simulink model "enabledSin"  (R2017a)
settings: Solver=VariableStepAuto  StartTime=0.0  StopTime=10.0  RelTol=1e-3
libraries: simulink x2
settings Model: Creator=eruffaldi  LastModifiedBy=eruffaldi

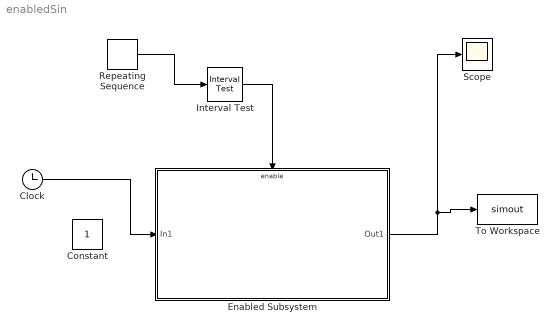
== system enabledSin ==
  Clock : Clock
  Constant : Constant
  Enabled Subsystem : Subsystem  TreatAsAtomicUnit=on
  Interval Test : simulink/Logic and Bit Operations/Interval Test  IntervalClosedRight=on  uplimit=3  IntervalClosedLeft=on  lowlimit=1  OutDataTypeStr=boolean
  Repeating Sequence : simulink/Sources/Repeating Sequence  rep_seq_t=[0 2 3]  rep_seq_y=[0 2 5]
  Scope : Scope
  To Workspace : ToWorkspace  VariableName=simout  SaveFormat=Timeseries  SampleTime=-1
  wires:
  Interval Test/1 -> Enabled Subsystem/Enable
  Repeating Sequence/1 -> Interval Test/1
  Enabled Subsystem/1(Out1) -> To Workspace/1, Scope/1
  Clock/1 -> Enabled Subsystem/1(In1)

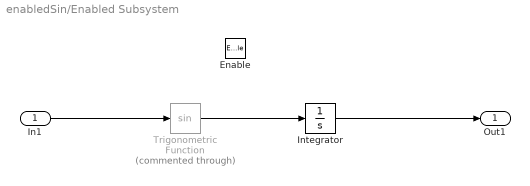
== system enabledSin/Enabled Subsystem ==
  In1 : Inport
  Enable : EnablePort  StatesWhenEnabling=reset
  Integrator : Integrator
  Trigonometric Function : Trigonometry  Commented=through
  Out1 : Outport  OutputWhenDisabled=reset  InitialOutput=[-1]
  wires:
  In1/1 -> Trigonometric Function/1
  Trigonometric Function/1 -> Integrator/1
  Integrator/1 -> Out1/1
